simulink model "Task8"  (R2023b)
settings: Solver=VariableStepAuto  StartTime=0.0  StopTime=10.0  RelTol=1e-3
values from neighbouring files (symbols this model uses):
  a = 0.5    [SYDE351Task8.m]    (also in task8.m)
  t_acc = V_max / a    (= 2)    [SYDE351Task8.m]    (also in task8.m)
  t_slew = 10    [SYDE351Task8.m]    (also in task8.m)
  V_max = 1.0    (= 1)    [SYDE351Task8.m]    (also in task8.m)
settings Model: Creator=bgonzalez  LastModifiedBy=bgonzalez

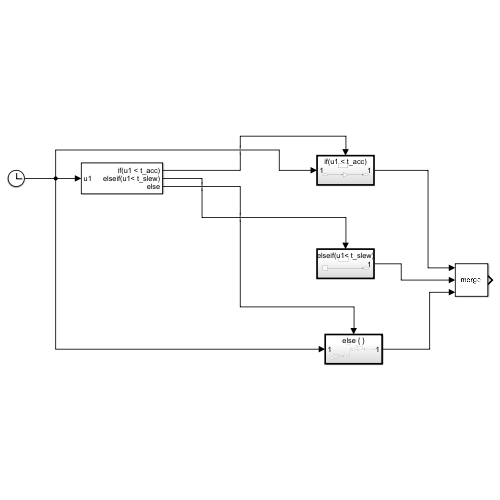
[thumbnail: Simulink's stored preview of the top-level diagram]
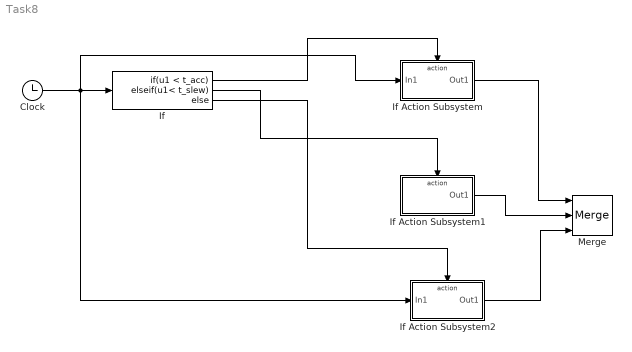
== system Task8 ==
  Clock : Clock
  If : If  IfExpression=u1 < t_acc  ElseIfExpressions=u1< t_slew
  If Action Subsystem : Subsystem  TreatAsAtomicUnit=on
  If Action Subsystem1 : Subsystem  TreatAsAtomicUnit=on
  If Action Subsystem2 : Subsystem  TreatAsAtomicUnit=on
  Merge : Merge  Inputs=3
  wires:
  Clock/1 -> If Action Subsystem2/1(In1), If Action Subsystem/1(In1), If/1
  If/1 -> If Action Subsystem/Action
  If/3 -> If Action Subsystem2/Action
  If Action Subsystem/1(Out1) -> Merge/1
  If Action Subsystem1/1(Out1) -> Merge/2
  If Action Subsystem2/1(Out1) -> Merge/3
  If/2 -> If Action Subsystem1/Action

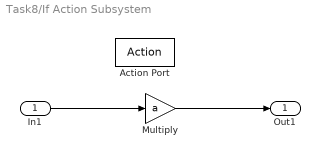
== system Task8/If Action Subsystem ==
  In1 : Inport
  Action Port : ActionPort  ActionPortLabel=if(u1 < t_acc)
  Multiply : Gain  Gain=a
  Out1 : Outport
  wires:
  In1/1 -> Multiply/1
  Multiply/1 -> Out1/1

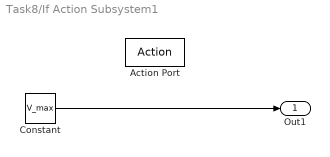
== system Task8/If Action Subsystem1 ==
  Action Port : ActionPort  ActionPortLabel=elseif(u1< t_slew)
  Constant : Constant  Value=V_max
  Out1 : Outport
  wires:
  Constant/1 -> Out1/1

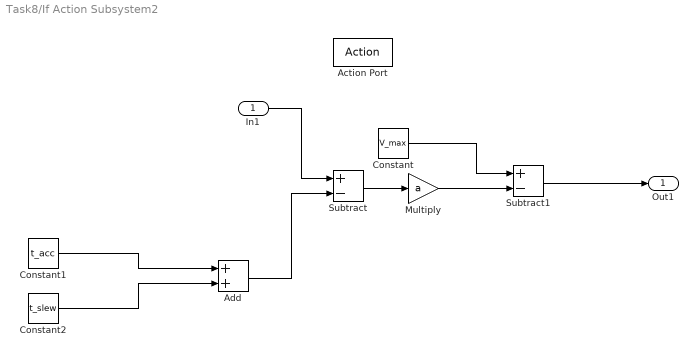
== system Task8/If Action Subsystem2 ==
  In1 : Inport
  Action Port : ActionPort  ActionPortLabel=else
  Add : Sum
  Constant : Constant  Value=V_max
  Constant1 : Constant  Value=t_acc
  Constant2 : Constant  Value=t_slew
  Multiply : Gain  Gain=a
  Subtract : Sum  Inputs=+-
  Subtract1 : Sum  Inputs=+-
  Out1 : Outport
  wires:
  Constant1/1 -> Add/1
  Constant2/1 -> Add/2
  In1/1 -> Subtract/1
  Add/1 -> Subtract/2
  Subtract/1 -> Multiply/1
  Multiply/1 -> Subtract1/2
  Constant/1 -> Subtract1/1
  Subtract1/1 -> Out1/1
